simulink model "Lab2_P2Q1c"  (R2019a)
settings: Solver=FixedStepDiscrete  StartTime=0.0  StopTime=10.0  FixedStep=0.01  RelTol=1e-3
settings Model: Creator=keeshigan  LastModifiedBy=keeshigan

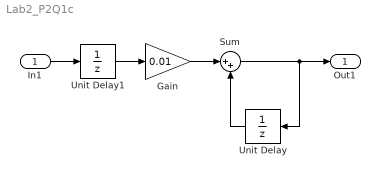
== system Lab2_P2Q1c ==
  In1 : Inport
  Gain : Gain  Gain=0.01
  Sum : Sum  Inputs=|++
  Unit Delay : UnitDelay  SampleTime=-1  HasFrameUpgradeWarning=on
  Unit Delay1 : UnitDelay  SampleTime=-1  HasFrameUpgradeWarning=on
  Out1 : Outport
  wires:
  Sum/1 -> Out1/1, Unit Delay/1
  Gain/1 -> Sum/1
  In1/1 -> Unit Delay1/1
  Unit Delay/1 -> Sum/2
  Unit Delay1/1 -> Gain/1
